simulink subsystem "barometer"  (R2024b)
settings: Solver=VariableStepAuto  StartTime=0.0  StopTime=10.0  RelTol=1e-3
undefined symbols (not defined in the file or in its folder): airdata, BARO_COV, BARO_RATE, GROUND_LEVEL, use_custom_atm
libraries: aerolibatmos2 x1
settings Model: Creator=yevge  LastModifiedBy=Aiden Gaydos

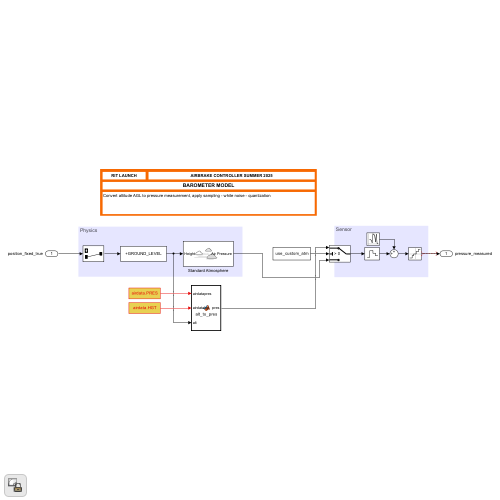
[thumbnail: Simulink's stored preview of the top-level diagram]
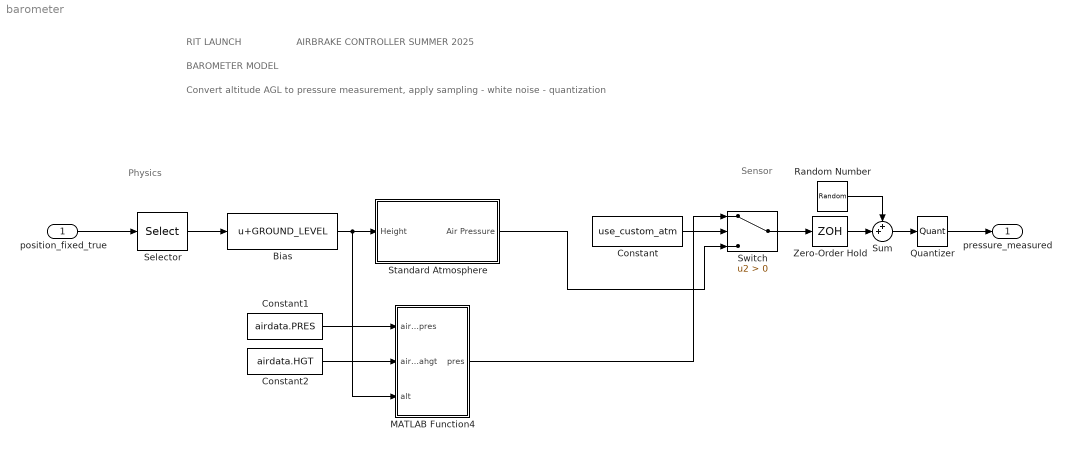
== system barometer ==
  note: Sensor
  note: Physics
  note: RIT LAUNCH
  note: BAROMETER MODEL
  note: Convert altitude AGL to pressure measurement, apply sampling - white noise - quantization
  note: AIRBRAKE CONTROLLER SUMMER 2025
  position_fixed_true : Inport  Unit=m  PortDimensions=[2 1]
  Bias : Bias  Bias=GROUND_LEVEL  SaturateOnIntegerOverflow=off
  Constant : Constant  Value=use_custom_atm
  Constant1 : Constant  Value=airdata.PRES
  Constant2 : Constant  Value=airdata.HGT
  MATLAB Function4 : MATLAB Function  TreatAsAtomicUnit=on
  Quantizer : Quantizer  QuantizationInterval=BARO_LSB
  Random Number : RandomNumber  Variance=BARO_COV  SampleTime=1/BARO_RATE
  Selector : Selector  InputPortWidth=2  IndexOptions=Index vector (dialog)  Indices=2  OutputSizes=1
  Standard Atmosphere : Subsystem
      mask Display:
      | block_icon("ISA Atmosphere Model")
      | 
      | % text(0.5 , 0.3, "ISA Pressure", ...
      | %     HorizontalAlignment="center", VerticalAlignment="middle")
      | % disp("\n\n\nISA Pressure");
  Sum : Sum  Inputs=++|
  Switch : Switch  Criteria=u2 > Threshold  SaturateOnIntegerOverflow=off  InputSameDT=off
  Zero-Order Hold : ZeroOrderHold  SampleTime=1/BARO_RATE
  pressure_measured : Outport  Unit=Pa  PortDimensions=1  SampleTime=1/BARO_RATE
  wires:
  position_fixed_true/1 -> Selector/1
  Selector/1 -> Bias/1
  ? -> ?
  Bias/1 -> Standard Atmosphere/1(Height), MATLAB Function4/3(alt)
  Zero-Order Hold/1 -> Sum/2
  Sum/1 -> Quantizer/1
  Random Number/1 -> Sum/1
  Quantizer/1 -> pressure_measured/1
  Constant1/1 -> MATLAB Function4/1(airdatapres)
  Constant2/1 -> MATLAB Function4/2(airdatahgt)
  Switch/1 -> Zero-Order Hold/1
  Constant/1 -> Switch/2
  Standard Atmosphere/1(Air Pressure) -> Switch/3
  MATLAB Function4/1(pres) -> Switch/1

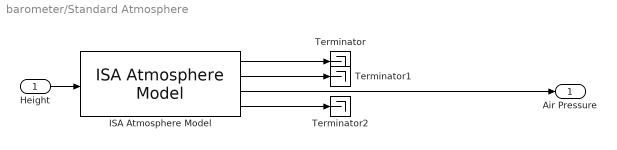
== system barometer/Standard Atmosphere ==
  Height : Inport
  ISA Atmosphere Model : aerolibatmos2/ISA Atmosphere Model  useExtended=off  action=Warning  custom=off  viscosityOut=off  g=9.80665  gamma=1.4  R=287.0531  L=0.0065  h_trop=11000  h_strat=20000  rho0=1.225  P0=101325  T0=288.15  h0=0  S=110.4  Tref=273.15  muref=1.716e-5
  Terminator : Terminator
  Terminator1 : Terminator
  Terminator2 : Terminator
  Air Pressure : Outport
  wires:
  Height/1 -> ISA Atmosphere Model/1
  ISA Atmosphere Model/4 -> Terminator2/1
  ISA Atmosphere Model/2 -> Terminator1/1
  ISA Atmosphere Model/3 -> Air Pressure/1
  ISA Atmosphere Model/1 -> Terminator/1

== matlab function barometer/MATLAB Function4 ==
  data: airdatapres input; airdatahgt input; alt input; pres output
function pres = alt_to_pres(airdatapres,airdatahgt,alt)
    pres = double(interp1(airdatahgt,airdatapres,alt,"linear","extrap"));
end
